simulink model "closed_loop"  (R2025b)
settings: Solver=VariableStepAuto  StartTime=0.0  StopTime=5.0  RelTol=1e-3
values from neighbouring files (symbols this model uses):
  A = [0 0 0 0 0 0 -4.52769230769 47.0088272383 1 0 -16.8834805098 55.3556738027 ... (16 elements, 4x4)]    [angle_sensor_data.mat]    (also in freq_experiments.m = [0, 0, 1, 0; inv_pend.m = [0, 0, 1, 0; lqr_tuning.m = [0, 0, 1, 0; position_sensor_data.mat)
  B = [0 0 3.77779700614 -12.3862196923]    [angle_sensor_data.mat]    (also in freq_experiments.m = [0; 0; (Km*Kg)/(M*Rm*r); (-Km*Kg)/(r*Rm*M*l)]; inv_pend.m = [0; 0; (Km*Kg)/(M*Rm*r); (-Km*Kg)/(r*Rm*M*l)]; lqr_tuning.m = [0; 0; (Km*Kg)/(M*Rm*r); (-Km*Kg)/(r*Rm*M*l)]; position_sensor_data.mat)
  K = [-18.2574185835 -93.1723220187 -24.9464299712 -21.1521187188]    [angle_sensor_data.mat]    (also in freq_experiments.m = lqr(A, B, Q, R); inv_pend.m = lqr(A, B, Q, R); lqr_tuning.m = lqr(A,B,Q,R); position_sensor_data.mat)
settings Model: Creator=sm  LastModifiedBy=sm

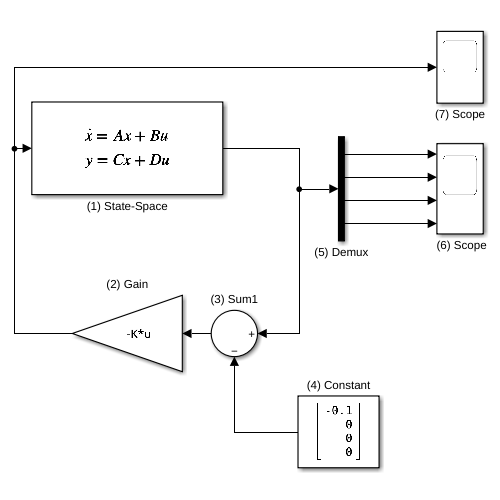
[thumbnail: Simulink's stored preview of the top-level diagram]
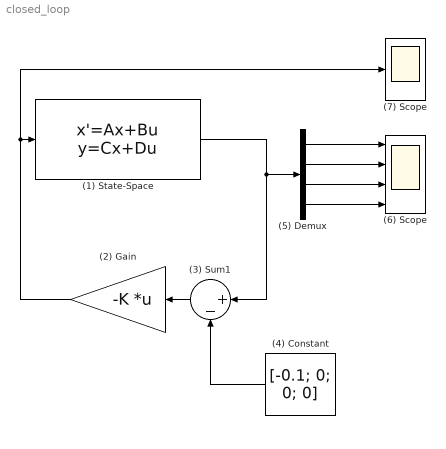
== system closed_loop ==
  " (6) Scope" : Scope  NumInputPorts=4
      settings: ActiveDisplayString=4  Title=Angular Velocity [rad/s]  ActiveDisplayYMinimum=-0.21748295419745842  ActiveDisplayYMaximum=0.072481637447331229
  (1) State-Space : StateSpace  A=A  B=B  C=eye(4)  D=zeros(4,1)  InitialCondition=[0; 0; 0; 0]
  (2) Gain : Gain  Gain=-K  Multiplication=Matrix(K*u)
  (3) Sum1 : Sum  Inputs=|+-
  (4) Constant : Constant  Value=[-0.1; 0; 0; 0]  VectorParams1D=off
  (5) Demux : Demux
  (7) Scope : Scope
      settings: Title=Control Input [V]  ActiveDisplayYMinimum=-0.4649296996377898  ActiveDisplayYMaximum=1.0659598879323
  wires:
  (5) Demux/4 -> " (6) Scope"/4
  (5) Demux/2 -> " (6) Scope"/2
  (5) Demux/1 -> " (6) Scope"/1
  (5) Demux/3 -> " (6) Scope"/3
  (1) State-Space/1 -> (3) Sum1/1, (5) Demux/1
  (2) Gain/1 -> (7) Scope/1, (1) State-Space/1
  (3) Sum1/1 -> (2) Gain/1
  (4) Constant/1 -> (3) Sum1/2
